simulink model "Model1"  (R2016a)
settings: Solver=VariableStepAuto  StartTime=0.0  StopTime=5.0  RelTol=1e-3
values from neighbouring files (symbols this model uses):
  J = 0.019    [parametriAM.m]    (also in podatki.m = 0.01)
  Lm = 0.0493    [parametriAM.m]    (also in podatki.m = 0.2342)
  Lr = 0.05315    [parametriAM.m]    (also in podatki.m = 0.2449)
  Ls = 0.05315    [parametriAM.m]    (also in podatki.m = 0.2449)
  pp = 3    [parametriAM.m]    (also in podatki.m = 2)
  Rs = 0.594    [parametriAM.m]    (also in podatki.m = 3.7)
  sigma = 1 - 1/((1+sigmaR)*(1+sigmaS))    (= 0.13962595434)    [parametriAM.m]
  Tr = Lr/Rr    (= 0.0771407837446)    [parametriAM.m]
undefined symbols (not defined in the file or in its folder): DiscIntNeverNeededParam
libraries: simulink x1
settings Model: Creator=Mitja1  LastModifiedBy=Mitja1

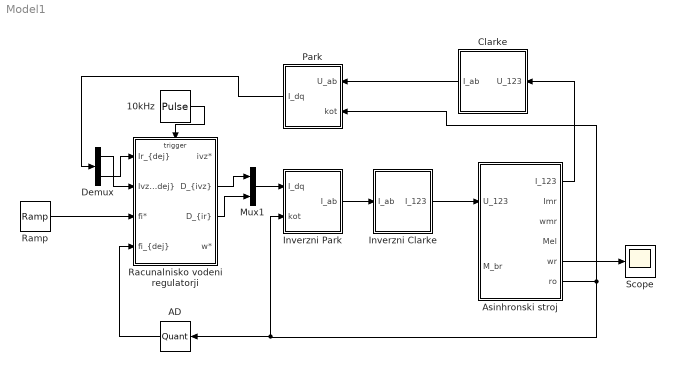
== system Model1 ==
  10kHz : DiscretePulseGenerator  PulseType=Time based  Period=1/10000  PulseWidth=5
  AD : Quantizer  QuantizationInterval=2*pi*2^-10
  Asinhronski stroj : Subsystem  InitFcn=parametriAM
  Clarke : Subsystem
  Demux : Demux  Outputs=2
  Inverzni Clarke : Subsystem
  Inverzni Park : Subsystem
  Mux1 : Mux  Inputs=2
  Park : Subsystem
  Racunalnisko vodeni regulatorji : Subsystem
  Ramp : simulink/Sources/Ramp  slope=90*2*pi/60  start=0.1  X0=0
  Scope : Scope
  wires:
  Inverzni Park/1(I_ab) -> Inverzni Clarke/1(I_ab)
  Inverzni Clarke/1(I_123) -> Asinhronski stroj/1(U_123)
  Asinhronski stroj/6(ro) -> Park/2(kot), AD/1, Inverzni Park/2(kot)
  Clarke/1(I_ab) -> Park/1(U_ab)
  Asinhronski stroj/1(I_123) -> Clarke/1(U_123)
  10kHz/1 -> Racunalnisko vodeni regulatorji/Trigger
  Mux1/1 -> Inverzni Park/1(I_dq)
  Racunalnisko vodeni regulatorji/2("D_{ivz}") -> Mux1/1
  Racunalnisko vodeni regulatorji/3("D_{ir}") -> Mux1/2
  Park/1(I_dq) -> Demux/1
  Demux/1 -> Racunalnisko vodeni regulatorji/2("Ivz_{dej}")
  Demux/2 -> Racunalnisko vodeni regulatorji/1("Ir_{dej}")
  Ramp/1 -> Racunalnisko vodeni regulatorji/3(fi*)
  AD/1 -> Racunalnisko vodeni regulatorji/4("fi_{dej}")
  Asinhronski stroj/5(wr) -> Scope/1

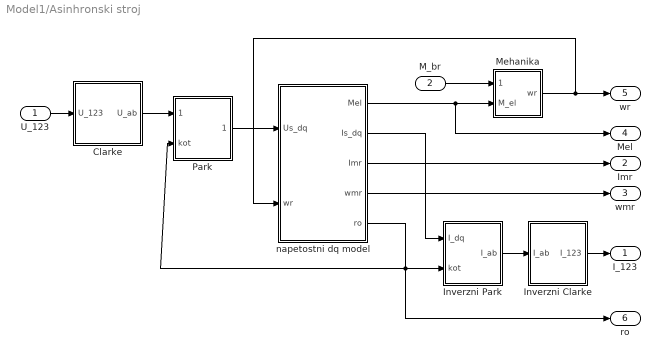
== system Model1/Asinhronski stroj ==
  U_123 : Inport
  M_br : Inport  Port=2
  Clarke : Subsystem
  Inverzni Clarke : Subsystem
  Inverzni Park : Subsystem
  Mehanika : Subsystem
  Park : Subsystem
  napetostni dq model : Subsystem
  I_123 : Outport
  Imr : Outport  Port=2
  wmr : Outport  Port=3
  Mel : Outport  Port=4
  wr : Outport  Port=5
  ro : Outport  Port=6
  wires:
  Inverzni Park/1(I_ab) -> Inverzni Clarke/1(I_ab)
  Clarke/1(U_ab) -> Park/1(U_ab)
  Mehanika/1(wr) -> napetostni dq model/2(wr), wr/1
  M_br/1 -> Mehanika/1(M_br)
  napetostni dq model/1(Mel) -> Mel/1, Mehanika/2(M_el)
  Inverzni Clarke/1(I_123) -> I_123/1
  napetostni dq model/4(wmr) -> wmr/1
  napetostni dq model/3(Imr) -> Imr/1
  U_123/1 -> Clarke/1(U_123)
  napetostni dq model/2(Is_dq) -> Inverzni Park/1(I_dq)
  napetostni dq model/5(ro) -> ro/1, Park/2(kot), Inverzni Park/2(kot)
  Park/1(U_dq) -> napetostni dq model/1(Us_dq)

== system Model1/Clarke ==
  U_123 : Inport
  ABC_ab1 : Subsystem
  Demux : Demux  Outputs=3
  Mux : Mux  Inputs=2
  I_ab : Outport
  wires:
  Mux/1 -> I_ab/1
  ABC_ab1/2(beta) -> Mux/2
  ABC_ab1/1(alfa) -> Mux/1
  Demux/3 -> ABC_ab1/3(C)
  Demux/2 -> ABC_ab1/2(B)
  Demux/1 -> ABC_ab1/1(A)
  U_123/1 -> Demux/1

== system Model1/Inverzni Clarke ==
  I_ab : Inport
  Demux : Demux  Outputs=2
  Mux : Mux  Inputs=3
  ab_ABC : Subsystem
  I_123 : Outport
  wires:
  ab_ABC/3(C) -> Mux/3
  ab_ABC/2(B) -> Mux/2
  ab_ABC/1(A) -> Mux/1
  Demux/2 -> ab_ABC/2(beta)
  Demux/1 -> ab_ABC/1(alfa)
  I_ab/1 -> Demux/1
  Mux/1 -> I_123/1

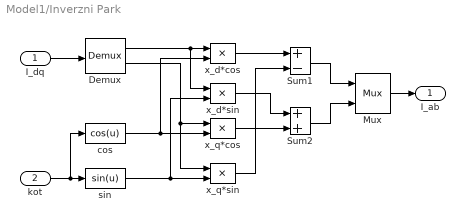
== system Model1/Inverzni Park ==
  I_dq : Inport
  kot : Inport  Port=2
  Demux : Demux  Outputs=2
  Mux : Mux  Inputs=2
  "Sum1 " : Sum  Inputs=+-  SaturateOnIntegerOverflow=on  InputSameDT=on  OutDataTypeStr=Inherit: Same as first input
  Sum2 : Sum  SaturateOnIntegerOverflow=on  InputSameDT=on  OutDataTypeStr=Inherit: Same as first input
  cos : Fcn  Expr=cos(u)
  sin : Fcn  Expr=sin(u)
  x_d*cos : Product  SaturateOnIntegerOverflow=on  RndMeth=Zero  InputSameDT=on  OutDataTypeStr=Inherit: Same as first input
  x_d*sin : Product  SaturateOnIntegerOverflow=on  RndMeth=Zero  InputSameDT=on  OutDataTypeStr=Inherit: Same as first input
  x_q*cos : Product  SaturateOnIntegerOverflow=on  RndMeth=Zero  InputSameDT=on  OutDataTypeStr=Inherit: Same as first input
  "x_q*sin " : Product  SaturateOnIntegerOverflow=on  RndMeth=Zero  InputSameDT=on  OutDataTypeStr=Inherit: Same as first input
  I_ab : Outport
  wires:
  Mux/1 -> I_ab/1
  I_dq/1 -> Demux/1
  Demux/1 -> x_d*sin/1, x_d*cos/1
  Demux/2 -> "x_q*sin "/1, x_q*cos/1
  cos/1 -> x_q*cos/2, x_d*cos/2
  sin/1 -> "x_q*sin "/2, x_d*sin/2
  x_d*cos/1 -> "Sum1 "/1
  "x_q*sin "/1 -> "Sum1 "/2
  x_q*cos/1 -> Sum2/2
  x_d*sin/1 -> Sum2/1
  "Sum1 "/1 -> Mux/1
  Sum2/1 -> Mux/2
  kot/1 -> cos/1, sin/1

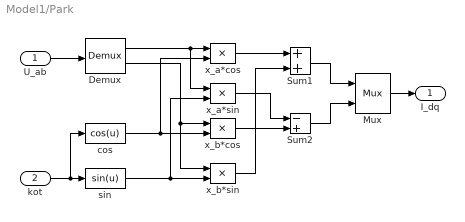
== system Model1/Park ==
  U_ab : Inport
  kot : Inport  Port=2
  Demux : Demux  Outputs=2
  Mux : Mux  Inputs=2
  "Sum1 " : Sum  SaturateOnIntegerOverflow=on  InputSameDT=on  OutDataTypeStr=Inherit: Same as first input
  Sum2 : Sum  Inputs=-+  SaturateOnIntegerOverflow=on  InputSameDT=on  OutDataTypeStr=Inherit: Same as first input
  cos : Fcn  Expr=cos(u)
  sin : Fcn  Expr=sin(u)
  x_a*cos : Product  SaturateOnIntegerOverflow=on  RndMeth=Zero  InputSameDT=on  OutDataTypeStr=Inherit: Same as first input
  x_a*sin : Product  SaturateOnIntegerOverflow=on  RndMeth=Zero  InputSameDT=on  OutDataTypeStr=Inherit: Same as first input
  x_b*cos : Product  SaturateOnIntegerOverflow=on  RndMeth=Zero  InputSameDT=on  OutDataTypeStr=Inherit: Same as first input
  "x_b*sin " : Product  SaturateOnIntegerOverflow=on  RndMeth=Zero  InputSameDT=on  OutDataTypeStr=Inherit: Same as first input
  I_dq : Outport
  wires:
  Mux/1 -> I_dq/1
  U_ab/1 -> Demux/1
  Demux/1 -> x_a*sin/1, x_a*cos/1
  Demux/2 -> "x_b*sin "/1, x_b*cos/1
  cos/1 -> x_b*cos/2, x_a*cos/2
  sin/1 -> "x_b*sin "/2, x_a*sin/2
  x_a*cos/1 -> "Sum1 "/1
  "x_b*sin "/1 -> "Sum1 "/2
  x_b*cos/1 -> Sum2/2
  x_a*sin/1 -> Sum2/1
  "Sum1 "/1 -> Mux/1
  Sum2/1 -> Mux/2
  kot/1 -> cos/1, sin/1

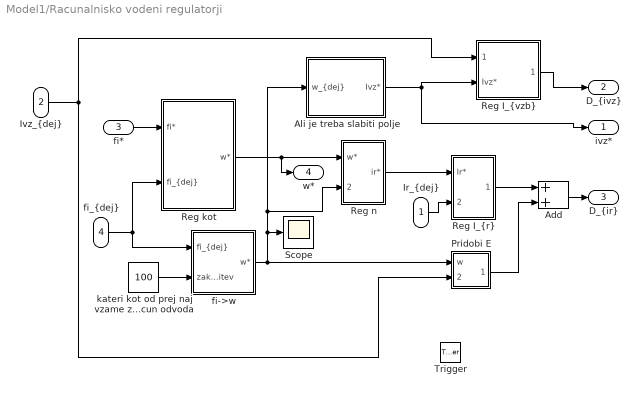
== system Model1/Racunalnisko vodeni regulatorji ==
  "Ir_{dej}" : Inport
  "Ivz_{dej}" : Inport  Port=2
  fi* : Inport  Port=3
  "fi_{dej}" : Inport  Port=4
  Trigger : TriggerPort  VariantControl=Variant  PortDimensions=1
  Add : Sum
  Ali je treba slabiti polje : Subsystem
  Pridobi E : Subsystem
  "Reg I_{r}" : Subsystem
  "Reg I_{vzb}" : Subsystem
  Reg kot : Subsystem
  Reg n : Subsystem
  Scope : Scope
  fi->w : Subsystem
  kateri kot od prej naj vzame za izracun odvoda : Constant  Value=100
  ivz* : Outport
  "D_{ivz}" : Outport  Port=2
  "D_{ir}" : Outport  Port=3
  w* : Outport  Port=4
  wires:
  fi*/1 -> Reg kot/1(fi*)
  kateri kot od prej naj vzame za izracun odvoda/1 -> fi->w/2(zakasnitev)
  "fi_{dej}"/1 -> Reg kot/2("fi_{dej}"), fi->w/1("fi_{dej}")
  fi->w/1(w*) -> Pridobi E/1(w), Reg n/2("w_{dej}"), Ali je treba slabiti polje/1("w_{dej} "), Scope/1
  "Ivz_{dej}"/1 -> Pridobi E/2(Ivz), "Reg I_{vzb}"/1("Ivz_{dej}")
  "Ir_{dej}"/1 -> "Reg I_{r}"/2("Ir_{dej}")
  Reg kot/1(w*) -> Reg n/1(w*), w*/1
  Pridobi E/1(~E/24) -> Add/2
  Ali je treba slabiti polje/1("Ivz* ") -> ivz*/1, "Reg I_{vzb}"/2(Ivz*)
  Add/1 -> "D_{ir}"/1
  "Reg I_{vzb}"/1("D_{ivz}") -> "D_{ivz}"/1
  Reg n/1(ir*) -> "Reg I_{r}"/1(Ir*)
  "Reg I_{r}"/1("D_{ir}") -> Add/1

== system Model1/Asinhronski stroj/Clarke ==
  U_123 : Inport
  ABC_ab1 : Subsystem
  Demux : Demux  Outputs=3
  Mux : Mux  Inputs=2
  U_ab : Outport
  wires:
  Mux/1 -> U_ab/1
  ABC_ab1/2(beta) -> Mux/2
  ABC_ab1/1(alfa) -> Mux/1
  Demux/3 -> ABC_ab1/3(C)
  Demux/2 -> ABC_ab1/2(B)
  Demux/1 -> ABC_ab1/1(A)
  U_123/1 -> Demux/1

== system Model1/Asinhronski stroj/Inverzni Clarke ==
  I_ab : Inport
  Demux : Demux  Outputs=2
  Mux : Mux  Inputs=3
  ab_ABC : Subsystem
  I_123 : Outport
  wires:
  ab_ABC/3(C) -> Mux/3
  ab_ABC/2(B) -> Mux/2
  ab_ABC/1(A) -> Mux/1
  Demux/2 -> ab_ABC/2(beta)
  Demux/1 -> ab_ABC/1(alfa)
  I_ab/1 -> Demux/1
  Mux/1 -> I_123/1

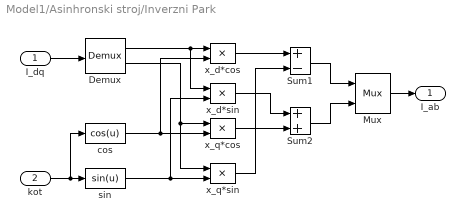
== system Model1/Asinhronski stroj/Inverzni Park ==
  I_dq : Inport
  kot : Inport  Port=2
  Demux : Demux  Outputs=2
  Mux : Mux  Inputs=2
  "Sum1 " : Sum  Inputs=+-  SaturateOnIntegerOverflow=on  InputSameDT=on  OutDataTypeStr=Inherit: Same as first input
  Sum2 : Sum  SaturateOnIntegerOverflow=on  InputSameDT=on  OutDataTypeStr=Inherit: Same as first input
  cos : Fcn  Expr=cos(u)
  sin : Fcn  Expr=sin(u)
  x_d*cos : Product  SaturateOnIntegerOverflow=on  RndMeth=Zero  InputSameDT=on  OutDataTypeStr=Inherit: Same as first input
  x_d*sin : Product  SaturateOnIntegerOverflow=on  RndMeth=Zero  InputSameDT=on  OutDataTypeStr=Inherit: Same as first input
  x_q*cos : Product  SaturateOnIntegerOverflow=on  RndMeth=Zero  InputSameDT=on  OutDataTypeStr=Inherit: Same as first input
  "x_q*sin " : Product  SaturateOnIntegerOverflow=on  RndMeth=Zero  InputSameDT=on  OutDataTypeStr=Inherit: Same as first input
  I_ab : Outport
  wires:
  Mux/1 -> I_ab/1
  I_dq/1 -> Demux/1
  Demux/1 -> x_d*sin/1, x_d*cos/1
  Demux/2 -> "x_q*sin "/1, x_q*cos/1
  cos/1 -> x_q*cos/2, x_d*cos/2
  sin/1 -> "x_q*sin "/2, x_d*sin/2
  x_d*cos/1 -> "Sum1 "/1
  "x_q*sin "/1 -> "Sum1 "/2
  x_q*cos/1 -> Sum2/2
  x_d*sin/1 -> Sum2/1
  "Sum1 "/1 -> Mux/1
  Sum2/1 -> Mux/2
  kot/1 -> cos/1, sin/1

== system Model1/Asinhronski stroj/Mehanika ==
  M_br : Inport
  M_el : Inport  Port=2
  Sum : Sum  Inputs=+-
  eq 2.19 : Subsystem
  wr : Outport
  wires:
  M_br/1 -> Sum/2
  Sum/1 -> eq 2.19/1(M)
  M_el/1 -> Sum/1
  eq 2.19/1(wr) -> wr/1

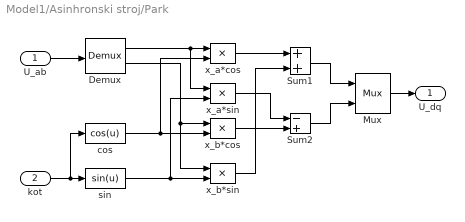
== system Model1/Asinhronski stroj/Park ==
  U_ab : Inport
  kot : Inport  Port=2
  Demux : Demux  Outputs=2
  Mux : Mux  Inputs=2
  "Sum1 " : Sum  SaturateOnIntegerOverflow=on  InputSameDT=on  OutDataTypeStr=Inherit: Same as first input
  Sum2 : Sum  Inputs=-+  SaturateOnIntegerOverflow=on  InputSameDT=on  OutDataTypeStr=Inherit: Same as first input
  cos : Fcn  Expr=cos(u)
  sin : Fcn  Expr=sin(u)
  x_a*cos : Product  SaturateOnIntegerOverflow=on  RndMeth=Zero  InputSameDT=on  OutDataTypeStr=Inherit: Same as first input
  x_a*sin : Product  SaturateOnIntegerOverflow=on  RndMeth=Zero  InputSameDT=on  OutDataTypeStr=Inherit: Same as first input
  x_b*cos : Product  SaturateOnIntegerOverflow=on  RndMeth=Zero  InputSameDT=on  OutDataTypeStr=Inherit: Same as first input
  "x_b*sin " : Product  SaturateOnIntegerOverflow=on  RndMeth=Zero  InputSameDT=on  OutDataTypeStr=Inherit: Same as first input
  U_dq : Outport
  wires:
  Mux/1 -> U_dq/1
  U_ab/1 -> Demux/1
  Demux/1 -> x_a*sin/1, x_a*cos/1
  Demux/2 -> "x_b*sin "/1, x_b*cos/1
  cos/1 -> x_b*cos/2, x_a*cos/2
  sin/1 -> "x_b*sin "/2, x_a*sin/2
  x_a*cos/1 -> "Sum1 "/1
  "x_b*sin "/1 -> "Sum1 "/2
  x_b*cos/1 -> Sum2/2
  x_a*sin/1 -> Sum2/1
  "Sum1 "/1 -> Mux/1
  Sum2/1 -> Mux/2
  kot/1 -> cos/1, sin/1

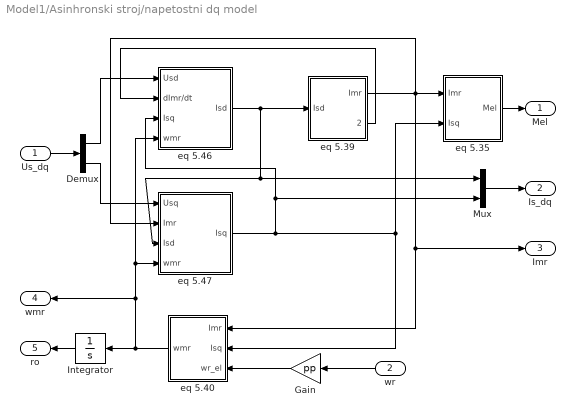
== system Model1/Asinhronski stroj/napetostni dq model ==
  Us_dq : Inport
  wr : Inport  Port=2
  Demux : Demux  Outputs=2
  Gain : Gain  Gain=pp
  Integrator : Integrator
  Mux : Mux  Inputs=2
  eq 5.35 : Subsystem
  eq 5.39 : Subsystem
  eq 5.40 : Subsystem
  eq 5.46 : Subsystem
  eq 5.47 : Subsystem
  Mel : Outport
  Is_dq : Outport  Port=2
  Imr : Outport  Port=3
  wmr : Outport  Port=4
  ro : Outport  Port=5
  wires:
  Gain/1 -> eq 5.40/3(wr_el)
  Mux/1 -> Is_dq/1
  Demux/2 -> eq 5.47/1(Usq)
  Demux/1 -> eq 5.46/1(Usd)
  Us_dq/1 -> Demux/1
  wr/1 -> Gain/1
  Integrator/1 -> ro/1
  eq 5.35/1(Mel) -> Mel/1
  eq 5.40/1(wmr) -> Integrator/1, wmr/1, eq 5.46/4(wmr), eq 5.47/4(wmr)
  eq 5.47/1(Isq) -> Mux/2, eq 5.46/3(Isq), eq 5.40/2(Isq), eq 5.35/2(Isq)
  eq 5.39/1(Imr) -> eq 5.47/2(Imr), Imr/1, eq 5.40/1(Imr), eq 5.35/1(Imr)
  eq 5.39/2(dImr/dt) -> eq 5.46/2(dImr/dt)
  eq 5.46/1(Isd) -> Mux/1, eq 5.47/3(Isd), eq 5.39/1(Isd)

== system Model1/Clarke/ABC_ab1 ==
  A : Inport
  B : Inport  Port=2
  C : Inport  Port=3
  Gain1 : Gain  Gain=2
  Gain2 : Gain
  Gain24 : Gain  Gain=sqrt(3)/3
  Sum11 : Sum
  Terminator : Terminator
  alfa : Outport
  beta : Outport  Port=2
  wires:
  C/1 -> Terminator/1
  Gain1/1 -> Sum11/2
  B/1 -> Gain1/1
  Gain24/1 -> beta/1
  Gain2/1 -> alfa/1
  Sum11/1 -> Gain24/1
  A/1 -> Sum11/1, Gain2/1

== system Model1/Inverzni Clarke/ab_ABC ==
  alfa : Inport
  beta : Inport  Port=2
  Gain1 : Gain
  Gain2 : Gain  Gain=-0.5
  Gain25 : Gain  Gain=sqrt(3)/2
  Gain3 : Gain  Gain=sqrt(3)/2
  Gain4 : Gain  Gain=0.5
  Sum10 : Sum
  Sum11 : Sum  Inputs=--
  A : Outport
  B : Outport  Port=2
  C : Outport  Port=3
  wires:
  Gain3/1 -> Sum11/2
  beta/1 -> Gain25/1, Gain3/1
  Gain4/1 -> Sum11/1
  Gain25/1 -> Sum10/2
  Gain2/1 -> Sum10/1
  alfa/1 -> Gain1/1, Gain2/1, Gain4/1
  Gain1/1 -> A/1
  Sum10/1 -> B/1
  Sum11/1 -> C/1

== system Model1/Racunalnisko vodeni regulatorji/Ali je treba slabiti polje ==
  "w_{dej} " : Inport
  Abs : Abs
  Add1 : Sum  Inputs=+-
  Constant : Constant  Value=24
  Constant1 : Constant  Value=2.66
  Divide : Product  Inputs=*/
  Gain : Gain  Gain=0.63
  Gain1 : Gain  Gain=2
  Gain2 : Gain  Gain=1.73
  Saturation : Saturate  UpperLimit=0.48  LowerLimit=0
  "Ivz* " : Outport
  wires:
  Constant1/1 -> Gain2/1
  Gain2/1 -> Gain1/1
  Constant/1 -> Add1/1
  Add1/1 -> Divide/1
  Gain/1 -> Divide/2
  "w_{dej} "/1 -> Gain/1
  Abs/1 -> Saturation/1
  Gain1/1 -> Add1/2
  Saturation/1 -> "Ivz* "/1
  Divide/1 -> Abs/1

== system Model1/Racunalnisko vodeni regulatorji/Pridobi E ==
  w : Inport
  Ivz : Inport  Port=2
  Divide : Product  Inputs=**
  Gain : Gain  Gain=0.63/24
  ~E/24 : Outport
  wires:
  Divide/1 -> Gain/1
  Ivz/1 -> Divide/1
  w/1 -> Divide/2
  Gain/1 -> ~E/24/1

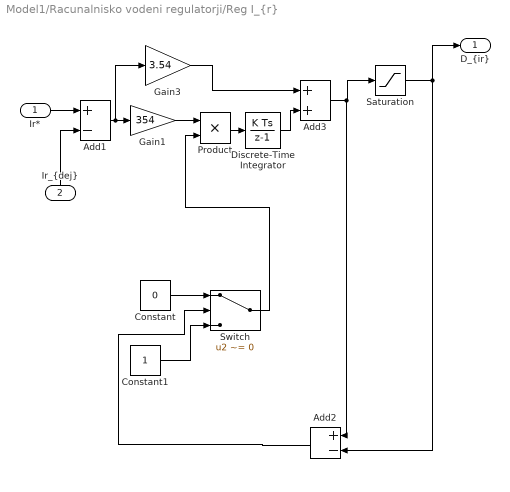
== system Model1/Racunalnisko vodeni regulatorji/Reg I_{r} ==
  Ir* : Inport
  "Ir_{dej}" : Inport  Port=2
  Add1 : Sum  Inputs=+-
  Add2 : Sum  Inputs=+-
  Add3 : Sum
  Constant : Constant  Value=0
  Constant1 : Constant
  Discrete-Time Integrator : DiscreteIntegrator  SampleTime=-1  ICPrevOutput=DiscIntNeverNeededParam  ICPrevScaledInput=DiscIntNeverNeededParam
  Gain1 : Gain  Gain=354
  Gain3 : Gain  Gain=3.54
  Product : Product
  Saturation : Saturate  UpperLimit=1  LowerLimit=-1
  Switch : Switch  Criteria=u2 ~= 0  ZeroCross=off
  "D_{ir}" : Outport
  wires:
  Product/1 -> Discrete-Time Integrator/1
  Gain1/1 -> Product/1
  Add2/1 -> Switch/2
  Constant1/1 -> Switch/3
  Constant/1 -> Switch/1
  Switch/1 -> Product/2
  Saturation/1 -> "D_{ir}"/1, Add2/2
  Add3/1 -> Saturation/1, Add2/1
  Ir*/1 -> Add1/1
  "Ir_{dej}"/1 -> Add1/2
  Add1/1 -> Gain3/1, Gain1/1
  Gain3/1 -> Add3/1
  Discrete-Time Integrator/1 -> Add3/2

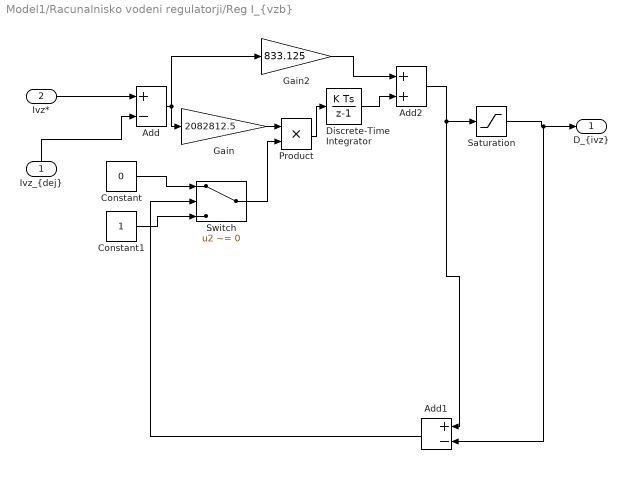
== system Model1/Racunalnisko vodeni regulatorji/Reg I_{vzb} ==
  "Ivz_{dej}" : Inport
  Ivz* : Inport  Port=2
  Add : Sum  Inputs=+-
  Add1 : Sum  Inputs=+-
  Add2 : Sum
  Constant : Constant  Value=0
  Constant1 : Constant
  Discrete-Time Integrator : DiscreteIntegrator  SampleTime=-1  ICPrevOutput=DiscIntNeverNeededParam  ICPrevScaledInput=DiscIntNeverNeededParam
  Gain : Gain  Gain=2082812.5
  Gain2 : Gain  Gain=833.125
  Product : Product
  Saturation : Saturate  UpperLimit=1  LowerLimit=-1
  Switch : Switch  Criteria=u2 ~= 0  ZeroCross=off
  "D_{ivz}" : Outport
  wires:
  Product/1 -> Discrete-Time Integrator/1
  Gain/1 -> Product/1
  Saturation/1 -> "D_{ivz}"/1, Add1/2
  Add1/1 -> Switch/2
  Constant1/1 -> Switch/3
  Constant/1 -> Switch/1
  Switch/1 -> Product/2
  Add2/1 -> Add1/1, Saturation/1
  "Ivz_{dej}"/1 -> Add/2
  Add/1 -> Gain2/1, Gain/1
  Ivz*/1 -> Add/1
  Gain2/1 -> Add2/1
  Discrete-Time Integrator/1 -> Add2/2

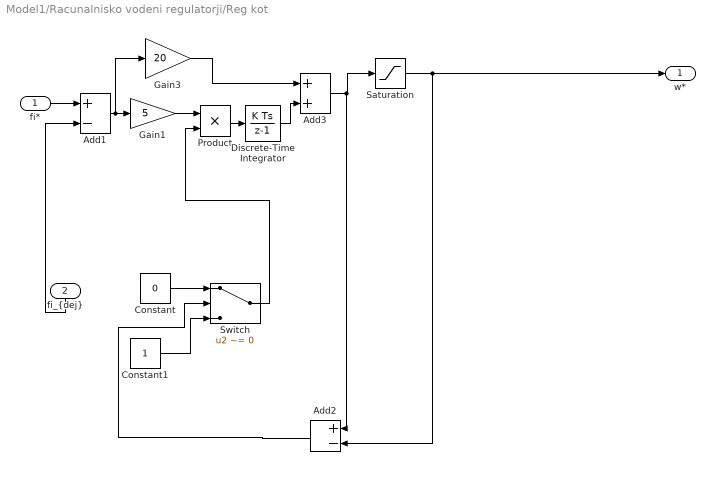
== system Model1/Racunalnisko vodeni regulatorji/Reg kot ==
  fi* : Inport
  "fi_{dej}" : Inport  Port=2
  Add1 : Sum  Inputs=+-
  Add2 : Sum  Inputs=+-
  Add3 : Sum
  Constant : Constant  Value=0
  Constant1 : Constant
  Discrete-Time Integrator : DiscreteIntegrator  SampleTime=-1  ICPrevOutput=DiscIntNeverNeededParam  ICPrevScaledInput=DiscIntNeverNeededParam
  Gain1 : Gain  Gain=5
  Gain3 : Gain  Gain=20
  Product : Product
  Saturation : Saturate  UpperLimit=1000*2*pi/60  LowerLimit=-1000*2*pi/60
  Switch : Switch  Criteria=u2 ~= 0  ZeroCross=off
  w* : Outport
  wires:
  Saturation/1 -> w*/1, Add2/2
  Product/1 -> Discrete-Time Integrator/1
  Gain1/1 -> Product/1
  Add2/1 -> Switch/2
  Constant1/1 -> Switch/3
  Constant/1 -> Switch/1
  Switch/1 -> Product/2
  Add3/1 -> Saturation/1, Add2/1
  fi*/1 -> Add1/1
  "fi_{dej}"/1 -> Add1/2
  Add1/1 -> Gain3/1, Gain1/1
  Gain3/1 -> Add3/1
  Discrete-Time Integrator/1 -> Add3/2

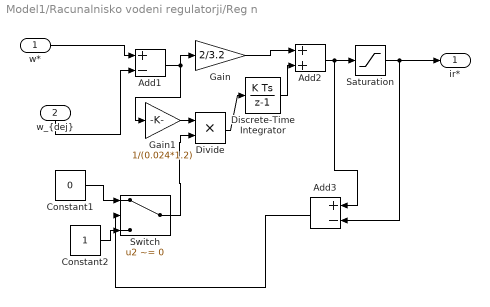
== system Model1/Racunalnisko vodeni regulatorji/Reg n ==
  w* : Inport
  "w_{dej}" : Inport  Port=2
  Add1 : Sum  Inputs=+-
  Add2 : Sum
  Add3 : Sum  Inputs=+-
  Constant1 : Constant  Value=0
  Constant2 : Constant
  Discrete-Time Integrator : DiscreteIntegrator  SampleTime=-1  ICPrevOutput=DiscIntNeverNeededParam  ICPrevScaledInput=DiscIntNeverNeededParam
  Divide : Product  Inputs=**
  Gain : Gain  Gain=2/3.2
  Gain1 : Gain  Gain=1/(0.024*1.2)
  Saturation : Saturate  UpperLimit=2.66  LowerLimit=-2.66
  Switch : Switch  Criteria=u2 ~= 0  ZeroCross=off
  ir* : Outport
  wires:
  Add3/1 -> Switch/2
  Constant2/1 -> Switch/3
  Constant1/1 -> Switch/1
  Switch/1 -> Divide/2
  Add2/1 -> Saturation/1, Add3/1
  Saturation/1 -> ir*/1, Add3/2
  Gain1/1 -> Divide/1
  Divide/1 -> Discrete-Time Integrator/1
  w*/1 -> Add1/1
  Discrete-Time Integrator/1 -> Add2/2
  Add1/1 -> Gain/1, Gain1/1
  Gain/1 -> Add2/1
  "w_{dej}"/1 -> Add1/2

== system Model1/Racunalnisko vodeni regulatorji/fi->w ==
  "fi_{dej}" : Inport
  zakasnitev : Inport  Port=2
  Delay1 : Delay  DelayLengthSource=Input port  DelayLength=10
      settings: InputPortMap=u0,p1
  Divide : Product  Inputs=*/
  Gain : Gain  Gain=10000
  Subtract : Sum  Inputs=+-
  w* : Outport
  wires:
  zakasnitev/1 -> Delay1/2, Divide/2
  Divide/1 -> Gain/1
  Gain/1 -> w*/1
  Delay1/1 -> Subtract/2
  Subtract/1 -> Divide/1
  "fi_{dej}"/1 -> Delay1/1, Subtract/1

== system Model1/Asinhronski stroj/Clarke/ABC_ab1 ==
  A : Inport
  B : Inport  Port=2
  C : Inport  Port=3
  Gain1 : Gain  Gain=2
  Gain2 : Gain
  Gain24 : Gain  Gain=sqrt(3)/3
  Sum11 : Sum
  Terminator : Terminator
  alfa : Outport
  beta : Outport  Port=2
  wires:
  C/1 -> Terminator/1
  Gain1/1 -> Sum11/2
  B/1 -> Gain1/1
  Gain24/1 -> beta/1
  Gain2/1 -> alfa/1
  Sum11/1 -> Gain24/1
  A/1 -> Sum11/1, Gain2/1

== system Model1/Asinhronski stroj/Inverzni Clarke/ab_ABC ==
  alfa : Inport
  beta : Inport  Port=2
  Gain1 : Gain
  Gain2 : Gain  Gain=-0.5
  Gain25 : Gain  Gain=sqrt(3)/2
  Gain3 : Gain  Gain=sqrt(3)/2
  Gain4 : Gain  Gain=0.5
  Sum10 : Sum
  Sum11 : Sum  Inputs=--
  A : Outport
  B : Outport  Port=2
  C : Outport  Port=3
  wires:
  Gain3/1 -> Sum11/2
  beta/1 -> Gain25/1, Gain3/1
  Gain4/1 -> Sum11/1
  Gain25/1 -> Sum10/2
  Gain2/1 -> Sum10/1
  alfa/1 -> Gain1/1, Gain2/1, Gain4/1
  Gain1/1 -> A/1
  Sum10/1 -> B/1
  Sum11/1 -> C/1

== system Model1/Asinhronski stroj/Mehanika/eq 2.19 ==
  M : Inport
  Gain1 : Gain  Gain=1/J
  Integrator : Integrator
  wr : Outport
  wires:
  Integrator/1 -> wr/1
  M/1 -> Gain1/1
  Gain1/1 -> Integrator/1

== system Model1/Asinhronski stroj/napetostni dq model/eq 5.35 ==
  Imr : Inport
  Isq : Inport  Port=2
  Gain : Gain  Gain=3*pp/2
  Gain2 : Gain  Gain=Lm*Lm/Lr
  Product : Product  RndMeth=Zero
  Mel : Outport
  wires:
  Gain/1 -> Gain2/1
  Gain2/1 -> Mel/1
  Product/1 -> Gain/1
  Isq/1 -> Product/2
  Imr/1 -> Product/1

== system Model1/Asinhronski stroj/napetostni dq model/eq 5.39 ==
  Isd : Inport
  Gain : Gain  Gain=1/Tr
  Integrator : Integrator  InitialCondition=1e-3
  Sum : Sum  Inputs=|+-
  Imr : Outport
  dImr/dt : Outport  Port=2
  wires:
  Gain/1 -> dImr/dt/1, Integrator/1
  Sum/1 -> Gain/1
  Integrator/1 -> Sum/2, Imr/1
  Isd/1 -> Sum/1

== system Model1/Asinhronski stroj/napetostni dq model/eq 5.40 ==
  Imr : Inport
  Isq : Inport  Port=2
  wr_el : Inport  Port=3
  Divide : Product  Inputs=*/
  Gain2 : Gain  Gain=Tr
  Saturation : Saturate  UpperLimit=2*pi*50  LowerLimit=-2*pi*50
  Sum : Sum  Inputs=|++
  wmr : Outport
  wires:
  Saturation/1 -> Sum/1
  Sum/1 -> wmr/1
  wr_el/1 -> Sum/2
  Divide/1 -> Saturation/1  "ws"
  Gain2/1 -> Divide/2
  Imr/1 -> Gain2/1
  Isq/1 -> Divide/1

== system Model1/Asinhronski stroj/napetostni dq model/eq 5.46 ==
  Usd : Inport
  dImr/dt : Inport  Port=2
  Isq : Inport  Port=3
  wmr : Inport  Port=4
  Gain : Gain  Gain=1/(sigma*Ls)
  Gain1 : Gain  Gain=Rs
  Gain2 : Gain  Gain=(1-sigma)*Ls
  Gain3 : Gain  Gain=sigma*Ls
  Integrator : Integrator
  Product : Product  RndMeth=Zero
  Sum : Sum  Inputs=+--+
  Isd : Outport
  wires:
  Gain3/1 -> Sum/4
  Product/1 -> Gain3/1
  Isq/1 -> Product/1
  wmr/1 -> Product/2
  Gain2/1 -> Sum/3
  dImr/dt/1 -> Gain2/1
  Gain1/1 -> Sum/2
  Usd/1 -> Sum/1
  Sum/1 -> Gain/1
  Gain/1 -> Integrator/1
  Integrator/1 -> Gain1/1, Isd/1

== system Model1/Asinhronski stroj/napetostni dq model/eq 5.47 ==
  Usq : Inport
  Imr : Inport  Port=2
  Isd : Inport  Port=3
  wmr : Inport  Port=4
  Gain : Gain  Gain=1/(sigma*Ls)
  Gain1 : Gain  Gain=Rs
  Gain2 : Gain  Gain=(1-sigma)*Ls
  Gain3 : Gain  Gain=sigma*Ls
  Integrator : Integrator
  Product : Product  RndMeth=Zero
  Product1 : Product  RndMeth=Zero
  Sum : Sum  Inputs=+---
  Isq : Outport
  wires:
  Gain3/1 -> Sum/4
  Product1/1 -> Gain3/1
  Isd/1 -> Product1/2
  Gain2/1 -> Sum/3
  Product/1 -> Gain2/1
  wmr/1 -> Product1/1, Product/2
  Imr/1 -> Product/1
  Gain1/1 -> Sum/2
  Usq/1 -> Sum/1
  Sum/1 -> Gain/1
  Gain/1 -> Integrator/1
  Integrator/1 -> Gain1/1, Isq/1
